simulink model "VEHICLE_DYN_TRAIN"  (R2019b)
settings: Solver=ode4  StartTime=0.0  StopTime=150  FixedStep=0.01  RelTol=1e-3
model workspace (MAT data in the model file):
  ACCEL = [0 0.000975932898663 -0.0414538855996 0.0440661905922 -0.0484817487001 0.0392964510644 -0.0693895143615 0.0261566921783 -0.0586295561215 0.0249771458914 -0.0595081132089 0.0233316013131 ... (544 elements, 17x32)]
  A_mc = 0.000491
  CMD_BR = [0 0 0 0 0 0 0 0 0 0 0 0 ... (15001 elements, 15001x1)]
  CMD_MODE = [1 1 1 1 1 1 1 1 1 1 1 1 ... (15001 elements, 15001x1)]
  CMD_ST = [0 0 0 0 0 0 0 0 0 0 0 0 ... (15001 elements, 15001x1)]
  CMD_T = [0 0.01 0.02 0.03 0.04 0.05 0.06 0.07 0.08 0.09 0.1 0.11 ... (2001 elements, 1x2001)]
  CMD_TH = [0 0 0 0 0 0 0 0 0 0 0 0 ... (15001 elements, 15001x1)]
  CMD_TM = [0 0.01 0.02 0.03 0.04 0.05 0.06 0.07 0.08 0.09 0.1 0.11 ... (15001 elements, 15001x1)]
  CMD_U = [10 10 10 10 10 10 10 10 10 10 10 10 ... (2001 elements, 1x2001)]
  CMD_UX = [0.1 0.1 0.1 0.1 0.1 0.1 0.1 0.1 0.1 0.1 0.1 0.1 ... (15001 elements, 15001x1)]
  COMMAND = [0 0 0 0 0 0 0 0 0 0 0 0 ... (102 elements, 17x6)]
  C_q = 1.4e-06
  DATA_HMMWV : object (value not decoded)
  DATA_VESIM_CC_BRAKE : object (value not decoded)
  FORCE = [0 -4628.45620853 2357.84853747 -1841.82564621 -1727.75397473 1695.19792057 -1263.06335256 1524.31841051 -1649.98396845 -1537.1025145 -1335.96213703 1639.88309903 ... (493 elements, 17x29)]
  F_cf = 80
  F_cs = 138
  F_z = -50097.6
  Gain_v = 70
  J_wheel = 32
  K_vb = 1500
  Kp_rpm = 2.7013
  Kp_v = 30
  L3 = 10
  MIN_TH = 0
  M_sprung = 4672
  M_unsprung = 220
  M_unsprung_front = 220
  M_vehicle = 5112
  N2 = 0
  N3 = 0.01
  P = 36
  P_0 = 10670
  P_gain = 0.0006
  R_wheel = 0.4412
  SLIP = [0 -0.5 0.5 -0.5 -0.5 0.5 -0.5 0.5 -0.5 -0.5 -0.5 0.5 ... (136 elements, 17x8)]
  STATE = [0 4.33747954961e-06 -0.000147430460781 -3.72129119222e-05 -0.000284189368187 -0.000207128204422 -0.00055150808757 -0.000594561033148 -0.000967775941564 -0.00103412952076 -0.00143215770154 -0.00152470872631 ... (544 elements, 17x32)]
  STATES_INIT = [0 0 0.9902452 0 0 1.57079632679 0.01 0 0 0 0 0 ... (32 elements, 1x32)]
  SUSP = [0 -0.00875795294893 -0.00878173856984 -0.00830852863719 -0.00873591176348 -0.00870428588158 -0.00751721170558 -0.00851904716693 -0.00789923296531 -0.00838039895253 -0.00756270047902 -0.00866403364289 ... (612 elements, 17x36)]
  S_o = 3
  T2_r = 4
  TIRE = [0 0.0910654620457 -0.0936729683319 0.0717372732987 0.0513932148365 -0.0365035701266 -0.00739813929507 -0.0045484168787 0.0723881675257 0.0296400174207 -0.0169805208571 0.0207214713062 ... (408 elements, 17x24)]
  TIRELIFTOFF = [0 0 0 0 0 0 0 0 0 0 0 0 ... (17 elements, 17x1)]
  T_LENGTH = 2001
  T_STEP = 0.01
  T_STOP = 12.82
  T_TOTAL = 20
  Ti_rpm = 0.6464
  Ti_v = 2.5
  Tstop = [150 150 150 150 150 150 150 150 150 150 150 150 ... (15001 elements, 15001x1)]
  Tt_rpm = 0.0808
  Tt_v = 0.3125
  U_INIT = 0.01
  b = 170
  brake_Pw = [-3.96235801772 -3.96238075942 -0.895107722214 -0.895547395081 35.9159438465 72.7273668629 152.485661058 244.514654481 330.408495385 364.152342142 462.316700341 535.939857177 ... (40 elements, 40x1)]
  brake_V = [-1.14468402636e-08 6.09303685082e-09 2.9257815427e-07 6.31682445149e-07 8.18779962309e-07 1.05849711081e-06 1.41515318379e-06 1.67826507702e-06 1.8361367918e-06 2.02323385108e-06 2.22788040303e-06 2.46760304614e-06 ... (40 elements, 40x1)]
  diff_efficiency = 0.94
  diff_wRatio = 6.052
  diff_w_ratio = 3.56
  end_time = 140
  engine_inertia = 0.53
  fmin_mg = [42.75 43.31 51.6 64.3 73.65 71.1 72.7 72.36]
  fmin_mg_na = [42.79 42.79 42.79 42.79 42.79 42.79 42.79 42.79]
  g = -9.8
  g_motor_eff = 1
  gr_motor = 0
  i = 5
  mdot_fuel = [5e-06 1e-05 2e-05 3e-05 4e-05 5e-05 6e-05 7e-05 8e-05]
  ms2mph = 2.23694
  n_tire = 4
  no_cyl = 8
  num_points = 14000
  num_points_fast = 140000
  rpm0 = 83.7758040957
  rpm0_c = 1000
  rpm2rads = 0.10471975512
  rpm_e = [50 800 1000 1500 2000 2500 3000 3300]
  rpm_engine = [700 800 1000 1500 2000 2500 3000 3300]
  rpm_hi_idle = 3400
  rpm_idle = 750
  rpm_max_c = 3200
  rpm_rated = 3200
  start_time = 0
  time_step = 0.01
  time_step_fast = 0.001
  torque_engine = [9.767 15.303 12.411 -4.524 -12.214 -35.77 -70 -75.889 75.383 80.318 76.501 61.314 ... (72 elements, 8x9)]
  tout = [0 0.01 0.02 0.03 0.04 0.05 0.06 0.07 0.08 0.09 0.1 0.11 ... (17 elements, 17x1)]
  trq_scale = 0.46
values from neighbouring files (symbols this model uses):
  B = Ref(i:i+2,2)    [Calc_vref.m]    (also in Parameter_load.m = 0.1; VEHICLE_DYN_TRAIN_INIT.m = 0.25)
  Error_now = Error_now_array(end)    [RUN_SIMULATION_SHARED_NEW_POWERTRAIN.m]    (also in VEHICLE_DYN_TRAIN_INIT.m = 0)
  J = 0.075    [VEHICLE_DYN_TRAIN_INIT.m]
  K = 0.075    [VEHICLE_DYN_TRAIN_INIT.m]
  pid2tau_gain = 2.5    [VEHICLE_DYN_TRAIN_INIT.m]
  st_a_in = st_sc_out(end)    [RUN_SIMULATION_SHARED_NEW_POWERTRAIN.m]    (also in VEHICLE_DYN_TRAIN_INIT.m = 0)
  tau_a_in = tau_a_out(end)    [RUN_SIMULATION_SHARED_NEW_POWERTRAIN.m]    (also in VEHICLE_DYN_TRAIN_INIT.m = 0)
undefined symbols (not defined in the file or in its folder): adaptive_flag, autonomy_human_contain_gain, Bias_Distance, dt, error_lookuptable, human_autonomy_agreement_threshold, human_contain_min, human_response_dead_zone, human_torque_max, J_cal, kp_sc, model_lookuptable, Standard_Devices, steering_stable_threshold, UDP_Protocol, vdes, Xobs, Yobs
libraries: simulink x16, sldrtlib x3, dspstat3 x3, vrlib x2
(part 2 of 4)

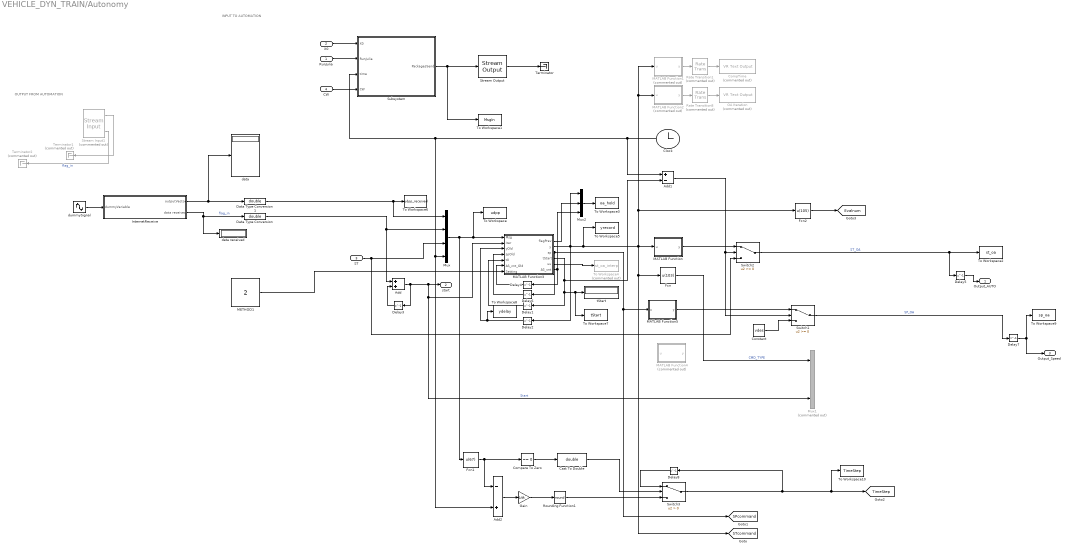
== system VEHICLE_DYN_TRAIN/Autonomy ==
  note: OUTPUT FROM AUTOMATION
  note: INPUT TO AUTOMATION
  RunJulia : Inport
  X0 : Inport  Port=2
  ST : Inport  Port=3
  CW : Inport  Port=4
  Add : Sum
  Add1 : Sum  Inputs=+-
  Add2 : Sum  Inputs=-+
  Cast To Double : DataTypeConversion  OutDataTypeStr=double
  Clock : Clock
      settings: Decimation=100
  CompTime : vrlib/VR Text Output  Commented=on  Ts=-1  ForceViewerOpen=off
      settings: SourceProductName=Simulink 3D Animation  SourceProductBaseCode=VR
  Compare To Zero : simulink/Logic and Bit Operations/Compare To Zero  relop===  OutDataTypeStr=boolean
  Constant : Constant  Value=vdes
  Data Type Conversion : DataTypeConversion  OutDataTypeStr=double
  Data Type Conversion1 : DataTypeConversion  OutDataTypeStr=double
  Delay{1,3..5,7..8} (6 alike) : Delay  DelayLength=1  InitialCondition=0  SampleTime=dt
  Delay2 : Delay  DelayLength=1  InitialCondition=zeros(110,1)  SampleTime=dt
  Delay6 : Delay  DelayLength=1  InitialCondition=zeros(110,1)  SampleTime=dt
  Fcn : Fcn  Expr=u(103)
  Fcn1 : Fcn  Expr=u(67)
  Fcn2 : Fcn  Expr=u(105)
  Gain : Gain  Gain=1/dt
  InternetReceive : Subsystem  mask(20-sim 4.6 S-Function block){}
      mask help:
      | This block is generated by the 20-sim Matlab Code Generator.
      |
      | * look under the mask to get information on the ports
      | * press Help for more detailed information
      | * the parameters of this block are:
      mask Help:
      | This block is generated by the 20-sim Matlab Code Generator<br>
      | The block parameters are:<br><blockquote></blockquote>
      | Generated at:<br>
      | <blockquote><b>date:  </b>June 14, 2017<br>
      | <b>time:  </b>4:16:43 PM<br></blockquote>
      | From the following 20-sim model:<br>
      | <blockquote><b>submodel:  </b>InternetServer<br>
      | <b>model:  </b>export to Simulink - UM<br>
      | <b>file:  </b>C:\Users\Tulga Ersal\Desktop\For Xueru\export to Simulink - UM.emx<br>
      | <b>experiment:  </b>C:\Users\Tulga Ersal\Desktop\For Xueru\export to Simulink - UM.emx<br></blockquote>
      | Using the following 20-sim license:<br>
      | <blockquote><b>user:  </b>The University of Michigan<br>
      | <b>from:  </b>20-sim 4.6 Student License<br>
      | <b>build: </b>4.6.1.6898<br></blockquote>
  MATLAB Function : MATLAB Function  TreatAsAtomicUnit=on
  MATLAB Function1 : MATLAB Function  Commented=on  TreatAsAtomicUnit=on
  MATLAB Function2 : MATLAB Function  Commented=on  TreatAsAtomicUnit=on
  MATLAB Function3 : MATLAB Function  TreatAsAtomicUnit=on
  MATLAB Function4 : MATLAB Function  Commented=on  TreatAsAtomicUnit=on
  MATLAB Function5 : MATLAB Function  TreatAsAtomicUnit=on
  METHOD1 : Constant  Value=2
  Mux : Mux
  Mux1 : Mux  Commented=on  Inputs=3
  Mux2 : Mux  Inputs=3
  OA Iteration : vrlib/VR Text Output  Commented=on  Ts=-1  ForceViewerOpen=off
      settings: SourceProductName=Simulink 3D Animation  SourceProductBaseCode=VR
  Rate Transition1 : RateTransition  Commented=on
  Rate Transition8 : RateTransition  Commented=on
  Rounding Function1 : Rounding  Operator=round
  Stream Input1 : sldrtlib/Stream Input  Commented=on  SampleTime=0.01  MaxMissedTicks=Inf  ShowMissedTicks=off  YieldWhenWaiting=off  DrvName=Standard_Devices/UDP_Protocol  DrvAddress=36881  DrvOptions=[0 12000 49 57 50 46 49 54 56 46 49 46 55 0 0 0 0 0 0 0 0 0 0 0 0 0 0 0 0 0 0 0 0 0 0 0 0 0 0 0 0 0 0 0 0 0 0 0 0 0 0 0 0 0 0 0 0 0 0 0 0 0 0 0 0 0 0 0 0 0 0 0 0 0 0 0 0 0 0 0 0 0 0 0 0 0 0 0 0 0 0 0 0 0 0 0 0 0 0 0 0 0 0 0 0 0 0 0 0 0 0 0 0 0 0 0 0 0 0 0 0 0 0 0 0 0 0 0 0 0 0 0 0 0 0 0 0 0 0 0 0 0 0 0 0 0 0 0 0 0 0 0 0 0 0 0 0 0 0 0 0 0 0 0 0 0 0 0 0 0 0 0 0 0 0 0 0 0 0 0 0 0 0 0 0 0 0 0 0 0 0 0 0 0 0 0 0 0 0 0 0 0 0 0 0 0 0 0 0 0 0 0 0 0 0 0 0 0 0 0 0 0 0 0 0 0 0 0 0 0 0 0 0 0 0 0 0 0 0 0 0 0 0 0 0 0 0 0 0 0 0 0 0 0 0 0]  DataTypes={'68*double'}  FormatString='%f,%f,%f,%f,%f,%f,%f,%f,%f,%f,%f,%f,%f,%f,%f,%f,%f,%f,%f,%f,%f,%f,%f,%f,%f,%f,%f,%f,%f,%f,%f,%f,%f,%f,%f,%f,%f,%f,%f,%f,%f,%f,%f,%f,%f,%f,%f,%f,%f,%f,%f,%f,%f,%f,%f,%f,%f,%f,%f,%f,%f,%f,%f,%f,%f,%f,%f,%f'  Terminator={ '\r', '\n' }  ShowReady=on  ShowError=off
      settings: AttributesFormatString=UDP Protocol [36881]  SourceProductName=Simulink Desktop Real-Time  SourceProductBaseCode=WT
  Stream Output : sldrtlib/Stream Output  SampleTime=0.01  MaxMissedTicks=Inf  ShowMissedTicks=on  YieldWhenWaiting=off  DrvName=Standard_Devices/UDP_Protocol  DrvAddress=36864  DrvOptions=[0 36880 49 57 50 46 49 54 56 46 49 46 55 0 0 0 0 0 0 0 0 0 0 0 0 0 0 0 0 0 0 0 0 0 0 0 0 0 0 0 0 0 0 0 0 0 0 0 0 0 0 0 0 0 0 0 0 0 0 0 0 0 0 0 0 0 0 0 0 0 0 0 0 0 0 0 0 0 0 0 0 0 0 0 0 0 0 0 0 0 0 0 0 0 0 0 0 0 0 0 0 0 0 0 0 0 0 0 0 0 0 0 0 0 0 0 0 0 0 0 0 0 0 0 0 0 0 0 0 0 0 0 0 0 0 0 0 0 0 0 0 0 0 0 0 0 0 0 0 0 0 0 0 0 0 0 0 0 0 0 0 0 0 0 0 0 0 0 0 0 0 0 0 0 0 0 0 0 0 0 0 0 0 0 0 0 0 0 0 0 0 0 0 0 0 0 0 0 0 0 0 0 0 0 0 0 0 0 0 0 0 0 0 0 0 0 0 0 0 0 0 0 0 0 0 0 0 0 0 0 0 0 0 0 0 0 0 0 0 0 0 0 0 0 0 0 0 0 0 0 0 0 0 0 0 0]  PortSizes=[23]  FormatString='%f %f %f %f %f %f %f %f %f %f %f %f %f %f %f %f %f %f %f %f %f %f %f \n'  ShowReady=off  ShowError=off  InitialValue=[]  FinalValue=[]
      settings: AttributesFormatString=UDP Protocol [36864]  SourceProductName=Simulink Desktop Real-Time  SourceProductBaseCode=WT
  Subsystem : Subsystem
  Switch1 : Switch
  Switch2 : Switch
  Switch3 : Switch  Criteria=u2 > Threshold
  Terminator : Terminator
  Terminator1 : Terminator  Commented=on
  Terminator2 : Terminator  Commented=on
  To Workspace : ToWorkspace  VariableName=udpp  SampleTime=-1
      settings: Save2DSignal=2-D array (concatenate along first dimension)
  To Workspace1 : ToWorkspace  VariableName=MsgIn  SampleTime=-1
  To Workspace10 : ToWorkspace  VariableName=TimeStep  SampleTime=-1
  To Workspace2 : ToWorkspace  VariableName=st_oa  SampleTime=-1
  To Workspace3 : ToWorkspace  VariableName=oa_hold  SampleTime=-1
  To Workspace4 : ToWorkspace  Commented=on  VariableName=st_oa_interp  SampleTime=-1
  To Workspace5 : ToWorkspace  VariableName=yrecord  SampleTime=-1
      settings: Save2DSignal=2-D array (concatenate along first dimension)
  To Workspace6 : ToWorkspace  VariableName=udpp_received  SampleTime=-1
      settings: Save2DSignal=2-D array (concatenate along first dimension)
  To Workspace7 : ToWorkspace  VariableName=tStart  SampleTime=-1
  To Workspace8 : ToWorkspace  VariableName=ydelay  SampleTime=-1
      settings: Save2DSignal=2-D array (concatenate along first dimension)
  To Workspace9 : ToWorkspace  VariableName=sp_oa  SampleTime=-1
  data : Display
  data received : Display
  dummySignal : Sin  SampleTime=0
  tStart : Display
  Output_AUTO : Outport  VectorParamsAs1DForOutWhenUnconnected=off
  start : Outport  Port=2  VectorParamsAs1DForOutWhenUnconnected=off
  Output_Speed : Outport  Port=3  VectorParamsAs1DForOutWhenUnconnected=off
  tag scope: Evalnum=global, SPcommand=global, STcommand=global, TimeStep=global
  wires:
  Data Type Conversion1/1 -> Mux/1, To Workspace6/1
  MATLAB Function3/5(uu) -> To Workspace4/1
  MATLAB Function/1(y) -> Switch2/1
  Add1/1 -> Switch1/2, Switch2/2
  Add/1 -> Delay3/1, Mux1/3, MATLAB Function3/2(iter), start/1  "Start"
  Subsystem/1(PackagesSend) -> Stream Output/1, To Workspace1/1
  Rate Transition8/1 -> OA Iteration/1
  MATLAB Function3/6(AS_cnt) -> Mux2/3, Delay4/1
  Fcn/1 -> Mux1/1  "CMD_TYPE"
  MATLAB Function2/1(y) -> Rate Transition8/1
  Rate Transition1/1 -> CompTime/1
  MATLAB Function3/4(tStart) -> Add1/2, Delay1/1, To Workspace7/1, tStart/1
  Delay4/1 -> MATLAB Function3/6(AS_cnt_Old)
  RunJulia/1 -> Subsystem/2(RunJulia)
  MATLAB Function3/1(flagPrev) -> Mux2/2
  Delay1/1 -> MATLAB Function3/5(t0)
  Data Type Conversion/1 -> Add/1, Mux/2
  Mux2/1 -> To Workspace3/1
  METHOD1/1 -> MATLAB Function3/7(Setting)
  Delay3/1 -> Add/2
  Switch2/1 -> Delay5/1, To Workspace2/1  "ST_OA"
  X0/1 -> Subsystem/1(X0)
  MATLAB Function1/1(y) -> Rate Transition1/1
  Delay2/1 -> To Workspace8/1, MATLAB Function3/3(yOld)
  Stream Output/1 -> Terminator/1
  ST/1 -> Switch2/3, Mux/3
  Delay5/1 -> Output_AUTO/1
  CW/1 -> Subsystem/4(CW)
  Delay6/1 -> MATLAB Function3/4(spOld)
  MATLAB Function5/1(y) -> Switch1/1
  Constant/1 -> Switch1/3
  Switch1/1 -> Delay7/1  "SP_OA"
  Delay7/1 -> Output_Speed/1, To Workspace9/1
  Delay8/1 -> Switch3/1
  Add2/1 -> Gain/1
  MATLAB Function3/3(sp) -> MATLAB Function5/1(u), [SPcommand], Delay6/1
  Cast To Double/1 -> Switch3/2
  Compare To Zero/1 -> Cast To Double/1
  Clock/1 -> Subsystem/3(time), Add2/2, Mux/4, Add1/1
  Mux/1 -> Fcn1/1, To Workspace/1, MATLAB Function3/1(Msg)
  Fcn1/1 -> Compare To Zero/1, Add2/1
  MATLAB Function3/2(y) -> Delay2/1, To Workspace5/1, [STcommand], Fcn/1, MATLAB Function1/1(u), MATLAB Function2/1(u), Fcn2/1, MATLAB Function/1(u), Mux2/1
  Fcn2/1 -> [Evalnum]
  Gain/1 -> Rounding Function1/1
  Rounding Function1/1 -> Switch3/3
  Switch3/1 -> [TimeStep], To Workspace10/1, Delay8/1
  InternetReceive/2(data received) -> Data Type Conversion/1, data received/1  "flag_in"
  dummySignal/1 -> InternetReceive/1(dummyVariable)
  InternetReceive/1(outputVector) -> Data Type Conversion1/1, data/1
  Stream Input1/1 -> Terminator1/1
  Stream Input1/2 -> Terminator2/1  "flag_in"

== system VEHICLE_DYN_TRAIN/Cognitive Workload Estimator ==
  Clock : Clock  Commented=on
  Constant : Constant
  Constant2 : Constant  Value=0.05
  Constant4 : Constant  Value=50
  Constant5 : Constant  Value=80
  MATLAB Function : MATLAB Function  Commented=on  TreatAsAtomicUnit=on
  Switch : Switch  Criteria=u2 > Threshold  Threshold=0.1
  Terminator : Terminator
  Workload : Outport  VectorParamsAs1DForOutWhenUnconnected=off
  wires:
  Clock/1 -> MATLAB Function/1(u)
  Constant2/1 -> Switch/2
  Constant5/1 -> Switch/1
  Constant4/1 -> Switch/3
  Switch/1 -> Workload/1
  Constant/1 -> Terminator/1

== system VEHICLE_DYN_TRAIN/Communication Unit ==
  HI : Inport
  Vehicle States : Inport  Port=2
  Speed : Inport  Port=3
  Demux : Demux
  Mux : Mux  Inputs=6
  Stream Output : sldrtlib/Stream Output  SampleTime=0.01  MaxMissedTicks=Inf  ShowMissedTicks=on  YieldWhenWaiting=off  DrvName=Standard_Devices/UDP_Protocol  DrvAddress=10001  DrvOptions=[0 10002 49 57 50 46 49 54 56 46 49 46 55 0 0 0 0 0 0 0 0 0 0 0 0 0 0 0 0 0 0 0 0 0 0 0 0 0 0 0 0 0 0 0 0 0 0 0 0 0 0 0 0 0 0 0 0 0 0 0 0 0 0 0 0 0 0 0 0 0 0 0 0 0 0 0 0 0 0 0 0 0 0 0 0 0 0 0 0 0 0 0 0 0 0 0 0 0 0 0 0 0 0 0 0 0 0 0 0 0 0 0 0 0 0 0 0 0 0 0 0 0 0 0 0 0 0 0 0 0 0 0 0 0 0 0 0 0 0 0 0 0 0 0 0 0 0 0 0 0 0 0 0 0 0 0 0 0 0 0 0 0 0 0 0 0 0 0 0 0 0 0 0 0 0 0 0 0 0 0 0 0 0 0 0 0 0 0 0 0 0 0 0 0 0 0 0 0 0 0 0 0 0 0 0 0 0 0 0 0 0 0 0 0 0 0 0 0 0 0 0 0 0 0 0 0 0 0 0 0 0 0 0 0 0 0 0 0 0 0 0 0 0 0 0 0 0 0 0 0 0 0 0 0 0 0]  PortSizes=[6]  FormatString='%f %f %f %f %f %f\n'  ShowReady=off  ShowError=off  InitialValue=[]  FinalValue=[]
      settings: AttributesFormatString=UDP Protocol [10001]  SourceProductName=Simulink Desktop Real-Time  SourceProductBaseCode=WT
  Terminator : Terminator
  wires:
  Stream Output/1 -> Terminator/1
  Demux/4 -> Mux/4
  Vehicle States/1 -> Demux/1
  Demux/3 -> Mux/3
  Demux/2 -> Mux/2
  Demux/1 -> Mux/1
  HI/1 -> Mux/5
  Mux/1 -> Stream Output/1
  Speed/1 -> Mux/6

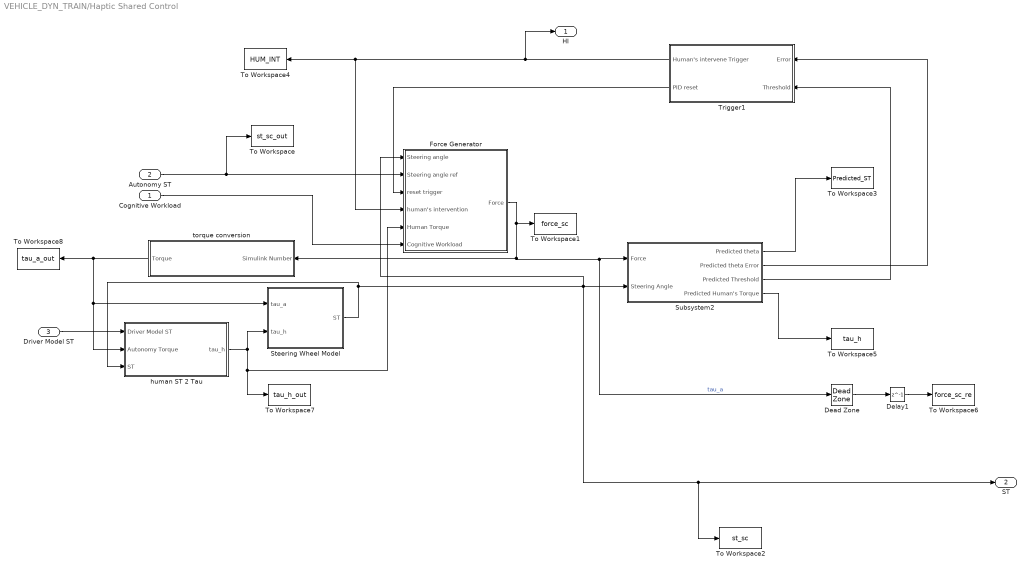
== system VEHICLE_DYN_TRAIN/Haptic Shared Control ==
  Cognitive Workload : Inport
  Autonomy ST : Inport  Port=2
  Driver Model ST : Inport  Port=3
  Dead Zone : DeadZone  LowerValue=F_f_n  UpperValue=F_f_p  SaturateOnIntegerOverflow=on
  Delay1 : Delay  DelayLength=1
  Force Generator : Subsystem
  Steering Wheel Model : Subsystem
  Subsystem2 : Subsystem
  To Workspace : ToWorkspace  VariableName=st_sc_out  SampleTime=-1
  To Workspace1 : ToWorkspace  VariableName=force_sc  SampleTime=-1
  To Workspace2 : ToWorkspace  VariableName=st_sc  SampleTime=-1
  To Workspace3 : ToWorkspace  VariableName=Predicted_ST  SampleTime=-1
  To Workspace4 : ToWorkspace  VariableName=HUM_INT  SampleTime=-1
  To Workspace5 : ToWorkspace  VariableName=tau_h  SampleTime=-1
  To Workspace6 : ToWorkspace  VariableName=force_sc_re  SampleTime=-1
  To Workspace7 : ToWorkspace  VariableName=tau_h_out  SampleTime=-1
  To Workspace8 : ToWorkspace  VariableName=tau_a_out  SampleTime=-1
  Trigger1 : Subsystem
  human ST 2 Tau : Subsystem
  torque conversion : Subsystem
  HI : Outport  VectorParamsAs1DForOutWhenUnconnected=off
  ST : Outport  Port=2  VectorParamsAs1DForOutWhenUnconnected=off
  wires:
  Subsystem2/1(Predicted theta) -> To Workspace3/1
  Cognitive Workload/1 -> Force Generator/6(Cognitive Workload)
  Trigger1/1(Human's intervene Trigger) -> HI/1, Force Generator/4(human's intervention), To Workspace4/1
  Subsystem2/2(Predicted theta Error) -> Trigger1/1(Error)
  Subsystem2/3(Predicted Threshold) -> Trigger1/2(Threshold)
  Trigger1/2(PID reset) -> Force Generator/3(reset trigger)
  Dead Zone/1 -> Delay1/1
  Subsystem2/4(Predicted Human's Torque) -> To Workspace5/1
  Delay1/1 -> To Workspace6/1
  Driver Model ST/1 -> human ST 2 Tau/1(Driver Model ST)
  Force Generator/1(Force) -> torque conversion/1(Simulink Number), Subsystem2/1(Force), Dead Zone/1, To Workspace1/1  "tau_a"
  Autonomy ST/1 -> To Workspace/1, Force Generator/2(Steering angle ref)
  torque conversion/1(Torque) -> human ST 2 Tau/2(Autonomy Torque), Steering Wheel Model/1(tau_a), To Workspace8/1
  human ST 2 Tau/1(tau_h) -> Force Generator/5(Human Torque), To Workspace7/1, Steering Wheel Model/2(tau_h)
  Steering Wheel Model/1(ST) -> human ST 2 Tau/3(ST), ST/1, To Workspace2/1, Subsystem2/2(Steering Angle), Force Generator/1(Steering angle)

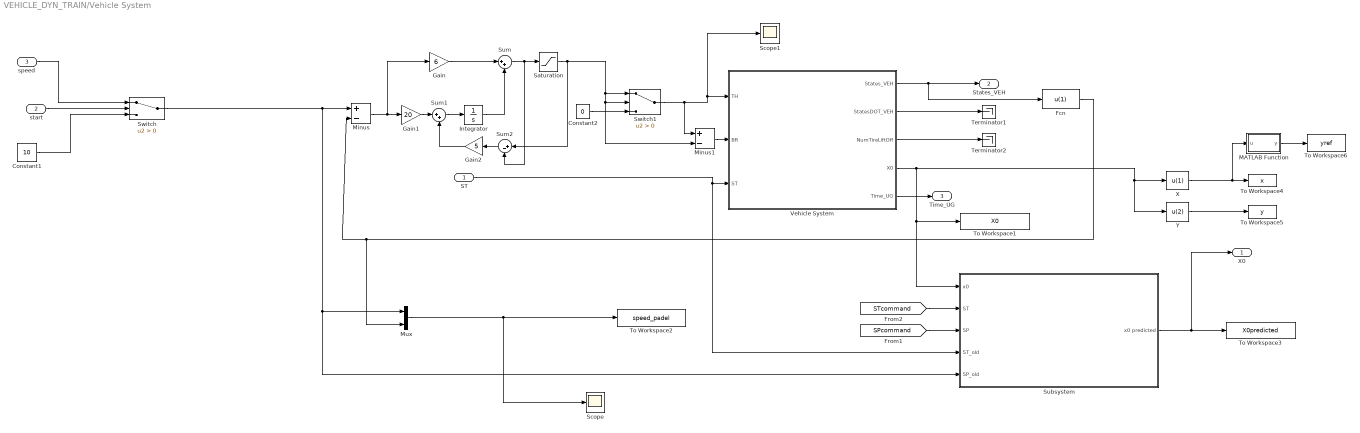
== system VEHICLE_DYN_TRAIN/Vehicle System ==
  ST : Inport
  start : Inport  Port=2
  speed : Inport  Port=3
  Constant1 : Constant  Value=10  SampleTime=dt
  Constant2 : Constant  Value=0  SampleTime=dt
  Fcn : Fcn  Expr=u(1)
  Gain : Gain  Gain=6
  Gain1 : Gain  Gain=20
  Gain2 : Gain  Gain=5
  Integrator : Integrator
  MATLAB Function : MATLAB Function  TreatAsAtomicUnit=on
  Minus : Sum  Inputs=+-
  Minus1 : Sum  Inputs=+-
  Mux : Mux  Inputs=2
  Saturation : Saturate  UpperLimit=1  LowerLimit=-1
  Scope : Scope
  Scope1 : Scope
  Subsystem : Subsystem
  Sum : Sum  Inputs=|++
  Sum1 : Sum  Inputs=|++
  Sum2 : Sum  Inputs=|+-
  Switch : Switch  Criteria=u2 > Threshold
  Switch1 : Switch  Criteria=u2 > Threshold
  Terminator1 : Terminator
  Terminator2 : Terminator
  To Workspace1 : ToWorkspace  VariableName=X0  SampleTime=-1
  To Workspace2 : ToWorkspace  VariableName=speed_padel  SampleTime=-1
  To Workspace3 : ToWorkspace  VariableName=X0predicted  SampleTime=-1
  To Workspace4 : ToWorkspace  VariableName=x  SampleTime=-1
  To Workspace5 : ToWorkspace  VariableName=y  SampleTime=-1
  To Workspace6 : ToWorkspace  VariableName=yref  SampleTime=-1
  Vehicle System : Subsystem
  X : Fcn  Expr=u(1)
  Y : Fcn  Expr=u(2)
  X0 : Outport  VectorParamsAs1DForOutWhenUnconnected=off
  States_VEH : Outport  Port=2  VectorParamsAs1DForOutWhenUnconnected=off
  Time_UG : Outport  Port=3  VectorParamsAs1DForOutWhenUnconnected=off
  wires:
  ST/1 -> Subsystem/4(ST_old), Vehicle System/3(ST)
  Vehicle System/1(States_VEH) -> Fcn/1, States_VEH/1
  Vehicle System/2(StatesDOT_VEH) -> Terminator1/1
  Vehicle System/3(NumTireLiftOff) -> Terminator2/1
  Fcn/1 -> Mux/2, Minus/2
  Minus/1 -> Gain1/1, Gain/1
  Gain/1 -> Sum/1
  Gain1/1 -> Sum1/1
  Sum1/1 -> Integrator/1
  Integrator/1 -> Sum/2
  Gain2/1 -> Sum1/2
  Sum2/1 -> Gain2/1
  Sum/1 -> Saturation/1, Sum2/2
  Saturation/1 -> Minus1/2, Switch1/2, Switch1/1, Sum2/1
  Switch1/1 -> Scope1/1, Vehicle System/1(TH), Minus1/1
  Constant2/1 -> Switch1/3
  Minus1/1 -> Vehicle System/2(BR)
  speed/1 -> Switch/1
  Constant1/1 -> Switch/3
  start/1 -> Switch/2
  Mux/1 -> Scope/1, To Workspace2/1
  Switch/1 -> Subsystem/5(SP_old), Mux/1, Minus/1
  [STcommand] -> Subsystem/2(ST)
  [SPcommand] -> Subsystem/3(SP)
  Subsystem/1(x0 predicted) -> X0/1, To Workspace3/1
  X/1 -> MATLAB Function/1(u), To Workspace4/1
  MATLAB Function/1(y) -> To Workspace6/1
  Y/1 -> To Workspace5/1
  Vehicle System/4(X0) -> Subsystem/1(x0), To Workspace1/1, Y/1, X/1
  Vehicle System/5(Time_UG) -> Time_UG/1

== system VEHICLE_DYN_TRAIN/Autonomy/InternetReceive ==
  dummyVariable : Inport
  Demux : Demux  Outputs=[1 -1]
  S-Function : S-Function  FunctionName=InternetServer  SFunctionDeploymentMode=off  EnableBusSupport=off
  outputVector : Outport  VectorParamsAs1DForOutWhenUnconnected=off
  data received : Outport  Port=2  VectorParamsAs1DForOutWhenUnconnected=off
  wires:
  dummyVariable/1 -> S-Function/1
  S-Function/1 -> Demux/1
  Demux/1 -> data received/1
  Demux/2 -> outputVector/1

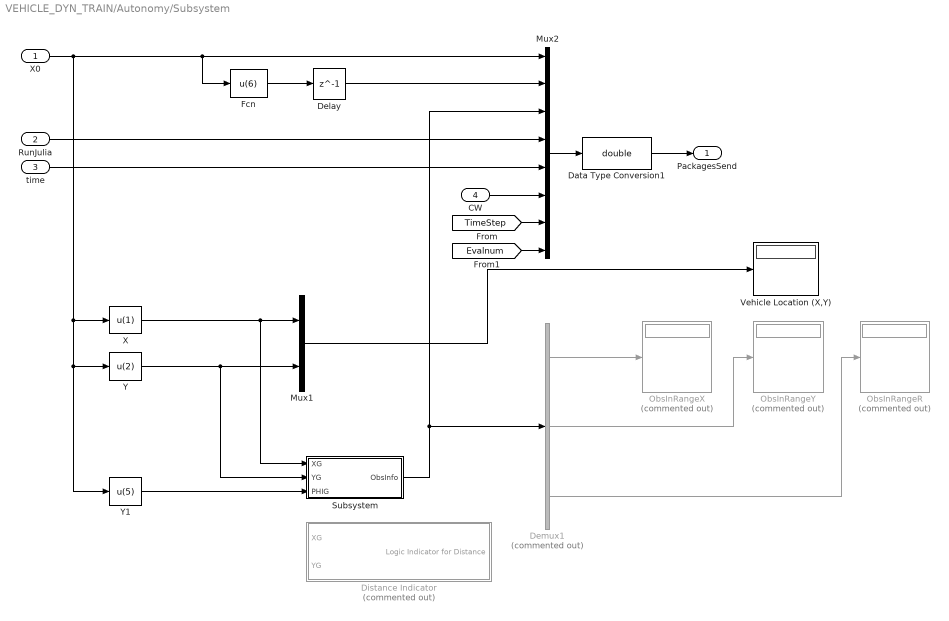
== system VEHICLE_DYN_TRAIN/Autonomy/Subsystem ==
  X0 : Inport
  RunJulia : Inport  Port=2
  time : Inport  Port=3
  CW : Inport  Port=4
  Data Type Conversion1 : DataTypeConversion  OutDataTypeStr=double
  Delay : Delay  DelayLength=1  InitialCondition=0  SampleTime=dt
  Demux1 : Demux  Commented=on  Outputs=[3 3 3]
  Distance Indicator : Subsystem  Commented=on
  Fcn : Fcn  Expr=u(6)
  Mux1 : Mux  Inputs=2
  Mux2 : Mux  Inputs=8
  ObsInRangeR : Display  Commented=on
  ObsInRangeX : Display  Commented=on
  ObsInRangeY : Display  Commented=on
  Subsystem : Subsystem
  Vehicle Location (X,Y) : Display
  X : Fcn  Expr=u(1)
  Y : Fcn  Expr=u(2)
  Y1 : Fcn  Expr=u(5)
  PackagesSend : Outport  VectorParamsAs1DForOutWhenUnconnected=off
  wires:
  Data Type Conversion1/1 -> PackagesSend/1
  Mux2/1 -> Data Type Conversion1/1
  X0/1 -> Y1/1, Y/1, X/1, Fcn/1, Mux2/1
  Y/1 -> Subsystem/2(YG), Mux1/2
  Subsystem/1(ObsInfo) -> Mux2/3, Demux1/1
  Mux1/1 -> Vehicle Location (X,Y)/1
  Demux1/1 -> ObsInRangeX/1
  Demux1/2 -> ObsInRangeY/1
  Demux1/3 -> ObsInRangeR/1
  time/1 -> Mux2/5
  RunJulia/1 -> Mux2/4
  Delay/1 -> Mux2/2
  Fcn/1 -> Delay/1
  Y1/1 -> Subsystem/3(PHIG)
  X/1 -> Subsystem/1(XG), Mux1/1
  CW/1 -> Mux2/6
  [TimeStep] -> Mux2/7
  [Evalnum] -> Mux2/8

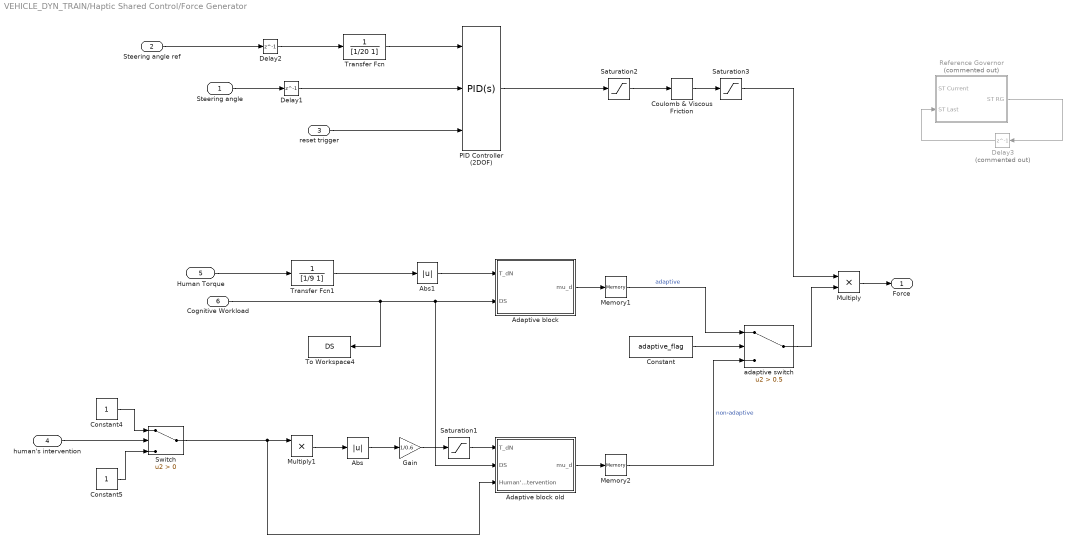
== system VEHICLE_DYN_TRAIN/Haptic Shared Control/Force Generator ==
  Steering angle : Inport
  Steering angle ref : Inport  Port=2
  reset trigger : Inport  Port=3
  human's intervention : Inport  Port=4
  Human Torque : Inport  Port=5
  Cognitive Workload : Inport  Port=6
  Abs : Abs
  Abs1 : Abs
  Adaptive block : Subsystem
  Adaptive block old : Subsystem
  Constant : Constant  Value=adaptive_flag
  Constant4 : Constant
  Constant5 : Constant
  Coulomb & Viscous Friction : simulink/Discontinuities/Coulomb & Viscous Friction  offset=0.12  gain=1
      settings: SourceProductName=Simulink
  Delay1 : Delay  DelayLength=1
  Delay2 : Delay  DelayLength=1
  Delay3 : Delay  Commented=on  DelayLength=1
  Gain : Gain  Gain=1/0.6
  Memory1 : Memory
  Memory2 : Memory
  Multiply : Product
  Multiply1 : Product
  PID Controller (2DOF) : simulink/Continuous/PID Controller (2DOF)  Controller=PID  Form=Parallel  TimeDomain=Continuous-time  SampleTime=-1  IntegratorMethod=Forward Euler  FilterMethod=Forward Euler  ControllerParametersSource=internal  P=20  I=10  D=0.75  UseFilter=on  N=100  b=1  c=1  TunerSelectOption=Transfer Function Based (PID Tuner App)  ZeroCross=off  InitialConditionSource=internal  InitialConditionForIntegrator=0  InitialConditionForFilter=0  DifferentiatorICPrevScaledInput=0  ExternalReset=rising  TrackingMode=off  Kt=1  LimitOutput=off  UpperSaturationLimit=inf  LowerSaturationLimit=-inf  LinearizeAsGain=on  AntiWindupMode=none  Kb=1  POutMin=[]  POutMax=[]  IOutMin=[]  IOutMax=[]  DOutMin=[]  DOutMax=[]  NOutMin=[]  NOutMax=[]  bOutMin=[]  bOutMax=[]  cOutMin=[]  cOutMax=[]  SumOutMin=[]  SumOutMax=[]  SaturationOutMin=[]  SaturationOutMax=[]  PParamMin=[]  PParamMax=[]  IParamMin=[]  IParamMax=[]  DParamMin=[]  DParamMax=[]  NParamMin=[]  NParamMax=[]  bParamMin=[]  bParamMax=[]  cParamMin=[]  cParamMax=[]  KbParamMin=[]  KbParamMax=[]  KtParamMin=[]  KtParamMax=[]  KbOutMin=[]  KbOutMax=[]  KtOutMin=[]  KtOutMax=[]  IntegratorOutMin=[]  IntegratorOutMax=[]  FilterOutMin=[]  FilterOutMax=[]  SumI1OutMin=[]  SumI1OutMax=[]  SumI2OutMin=[]  SumI2OutMax=[]  SumI3OutMin=[]  SumI3OutMax=[]  SumI4OutMin=[]  SumI4OutMax=[]  SumDOutMin=[]  SumDOutMax=[]  Sum1OutMin=[]  Sum1OutMax=[]  Sum2OutMin=[]  Sum2OutMax=[]  Sum3OutMin=[]  Sum3OutMax=[]  DifferentiatorOutMin=[]  DifferentiatorOutMax=[]  FilterDiffOutCoefMin=[]  FilterDiffOutCoefMax=[]  ReciprocalOutMin=[]  ReciprocalOutMax=[]  SumDenOutMin=[]  SumDenOutMax=[]  SumNumOutMin=[]  SumNumOutMax=[]  DivideOutMin=[]  DivideOutMax=[]  IntegratorContinuousStateAttributes=''  IntegratorStateMustResolveToSignalObject=off  IntegratorRTWStateStorageClass=Auto  FilterContinuousStateAttributes=''  FilterStateMustResolveToSignalObject=off  FilterRTWStateStorageClass=Auto  ParallelPVariant=InternalParameters  IdealPVariant=Disabled  IVariant=InternalParameters  DVariant=InternalParameters  bVariant=InternalParameters  cVariant=InternalParameters  IntegratorVariant=Continuous  SatVariant=Disabled  AWVariant=Passthrough  PCopyVariant=Disabled  TRVariant=Disabled  FdbkBlocksVariant=Forward  IdealPFdbkVariant=Disabled  SatFdbkVariant=Disabled  DerivativeFilterVariant=ContFilter  NVariant=InternalParameters  NCopyVariant=Disabled  FilterICVariant=InternalICsFilter  IntegratorICVariant=InternalICs  ExternalResetVariant=ExternalReset  TRSumVariant=Passthrough  SumFdbkVariant=Disabled  SumVariant=Sum_PID
  Reference Governor : Subsystem  Commented=on
  Saturation1 : Saturate  UpperLimit=1  LowerLimit=0
  Saturation2 : Saturate  UpperLimit=0.59  LowerLimit=-0.59
  Saturation3 : Saturate  UpperLimit=0.59  LowerLimit=-0.59
  Switch : Switch  Criteria=u2 > Threshold
  To Workspace4 : ToWorkspace  VariableName=DS  SampleTime=-1
  Transfer Fcn : TransferFcn  Denominator=[1/20 1]
  Transfer Fcn1 : TransferFcn  Denominator=[1/9 1]
  adaptive switch : Switch  Criteria=u2 > Threshold  Threshold=0.5
  Force : Outport  VectorParamsAs1DForOutWhenUnconnected=off
  wires:
  Steering angle/1 -> Delay1/1
  Delay1/1 -> PID Controller (2DOF)/2
  Saturation2/1 -> Coulomb & Viscous Friction/1
  PID Controller (2DOF)/1 -> Saturation2/1
  Coulomb & Viscous Friction/1 -> Saturation3/1
  Steering angle ref/1 -> Delay2/1
  Saturation3/1 -> Multiply/1
  Multiply/1 -> Force/1
  Adaptive block old/1(mu_d) -> Memory2/1
  Gain/1 -> Saturation1/1
  Abs/1 -> Gain/1
  Saturation1/1 -> Adaptive block old/1(T_dN)
  Switch/1 -> Adaptive block old/3(Human's intervention), Multiply1/1
  Multiply1/1 -> Abs/1
  reset trigger/1 -> PID Controller (2DOF)/3
  Reference Governor/1(ST RG) -> Delay3/1
  Delay3/1 -> Reference Governor/2(ST Last)
  Delay2/1 -> Transfer Fcn/1
  Transfer Fcn/1 -> PID Controller (2DOF)/1
  Constant4/1 -> Switch/1
  Constant5/1 -> Switch/3
  human's intervention/1 -> Switch/2
  Adaptive block/1(mu_d) -> Memory1/1
  Cognitive Workload/1 -> To Workspace4/1, Adaptive block old/2(DS), Adaptive block/2(DS)
  Abs1/1 -> Adaptive block/1(T_dN)
  Human Torque/1 -> Transfer Fcn1/1
  Memory1/1 -> adaptive switch/1  "adaptive"
  Memory2/1 -> adaptive switch/3  "non-adaptive"
  Transfer Fcn1/1 -> Abs1/1
  adaptive switch/1 -> Multiply/2
  Constant/1 -> adaptive switch/2

== system VEHICLE_DYN_TRAIN/Haptic Shared Control/Steering Wheel Model ==
  tau_a : Inport
  tau_h : Inport  Port=2
  Constant : Constant  Value=0
  Drag1 : Gain  Gain=B
  Gain : Gain  Gain=0.1
  Integrator1 : Integrator
  Integrator2 : Integrator
  Moment of Inertia1 : Gain  Gain=1/J
  Stiffness : Gain  Gain=K
  Sum : Sum  Inputs=|++
  Sum3 : Sum  Inputs=|+-
  Sum5 : Sum  Inputs=|++
  Terminator : Terminator
  ST : Outport  VectorParamsAs1DForOutWhenUnconnected=off
  wires:
  Sum/1 -> Sum3/1  "tau_in"
  Sum5/1 -> Sum3/2
  Drag1/1 -> Sum5/1
  Integrator2/1 -> Stiffness/1, Gain/1  "theta"
  Integrator1/1 -> Drag1/1, Integrator2/1  "omega"
  Moment of Inertia1/1 -> Integrator1/1  "omega_dot"
  Sum3/1 -> Moment of Inertia1/1
  Stiffness/1 -> Sum5/2
  Gain/1 -> ST/1
  tau_a/1 -> Sum/2  "tau_a"
  Constant/1 -> Terminator/1
  tau_h/1 -> Sum/1

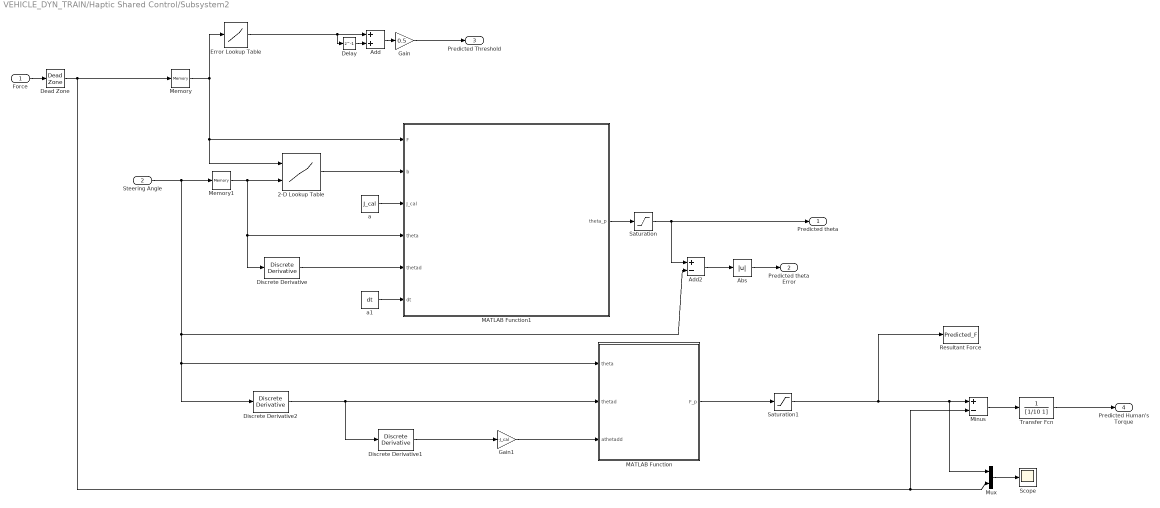
== system VEHICLE_DYN_TRAIN/Haptic Shared Control/Subsystem2 ==
  Force : Inport
  Steering Angle : Inport  Port=2
  2-D Lookup Table : Lookup_n-D  BreakpointsForDimension1=model_lookuptable.Breakpoints_row  BreakpointsForDimension2=model_lookuptable.Breakpoints_column  Table=model_lookuptable.Tabledata  InternalRulePriority=Speed  RndMeth=Simplest  InputSameDT=on
  Abs : Abs
  Add : Sum
  Add2 : Sum  Inputs=+-
  Dead Zone : DeadZone  LowerValue=F_f_n  UpperValue=F_f_p  SaturateOnIntegerOverflow=on
  Delay : Delay  DelayLength=1
  Discrete Derivative : simulink/Discrete/Discrete Derivative  gainval=1.0  ICPrevScaledInput=0.0  OutMin=[]  OutMax=[]  OutDataType=fixdt(1, 16)  OutScaling=2^-10  DoSatur=off
  Discrete Derivative1 : simulink/Discrete/Discrete Derivative  gainval=1.0  ICPrevScaledInput=0.0  OutMin=[]  OutMax=[]  OutDataType=fixdt(1, 16)  OutScaling=2^-10  DoSatur=off
  Discrete Derivative2 : simulink/Discrete/Discrete Derivative  gainval=1.0  ICPrevScaledInput=0.0  OutMin=[]  OutMax=[]  OutDataType=fixdt(1, 16)  OutScaling=2^-10  DoSatur=off
  Error Lookup Table : Lookup_n-D  NumberOfTableDimensions=1  BreakpointsForDimension1=error_lookuptable.Breakpoints  Table=error_lookuptable.Tabledata  InternalRulePriority=Speed  RndMeth=Simplest  InputSameDT=on
  Gain : Gain  Gain=0.5
  Gain1 : Gain  Gain=-J_cal
  MATLAB Function : MATLAB Function  TreatAsAtomicUnit=on
  MATLAB Function1 : MATLAB Function  TreatAsAtomicUnit=on
  Memory : Memory
  Memory1 : Memory
  Minus : Sum  Inputs=+-
  Mux : Mux  Inputs=2
  Resultant Force : ToWorkspace  VariableName=Predicted_F  SampleTime=-1
  Saturation : Saturate  UpperLimit=9/180*pi  LowerLimit=-9/180*pi
  Saturation1 : Saturate  UpperLimit=0.4386  LowerLimit=-0.4228
  Scope : Scope
  Transfer Fcn : TransferFcn  Denominator=[1/10 1]
  a : Constant  Value=J_cal
  a1 : Constant  Value=dt
  Predicted theta : Outport  VectorParamsAs1DForOutWhenUnconnected=off
  Predicted theta Error : Outport  Port=2  VectorParamsAs1DForOutWhenUnconnected=off
  Predicted Threshold : Outport  Port=3  VectorParamsAs1DForOutWhenUnconnected=off
  Predicted Human's Torque : Outport  Port=4  VectorParamsAs1DForOutWhenUnconnected=off
  wires:
  Discrete Derivative/1 -> MATLAB Function1/5(thetad)
  Saturation/1 -> Add2/1, Predicted theta/1
  Discrete Derivative1/1 -> Gain1/1
  Force/1 -> Dead Zone/1
  Gain1/1 -> MATLAB Function/3(athetadd)
  MATLAB Function/1(F_p) -> Saturation1/1
  Saturation1/1 -> Mux/1, Minus/1, Resultant Force/1
  Add2/1 -> Abs/1
  Abs/1 -> Predicted theta Error/1
  a/1 -> MATLAB Function1/3(J_cal)
  2-D Lookup Table/1 -> MATLAB Function1/2(b)
  MATLAB Function1/1(theta_p) -> Saturation/1
  a1/1 -> MATLAB Function1/6(dt)
  Steering Angle/1 -> Memory1/1, Add2/2, MATLAB Function/1(theta), Discrete Derivative2/1
  Memory/1 -> MATLAB Function1/1(F), 2-D Lookup Table/1, Error Lookup Table/1
  Memory1/1 -> Discrete Derivative/1, MATLAB Function1/4(theta), 2-D Lookup Table/2
  Discrete Derivative2/1 -> Discrete Derivative1/1, MATLAB Function/2(thetad)
  Delay/1 -> Add/2
  Error Lookup Table/1 -> Delay/1, Add/1
  Add/1 -> Gain/1
  Gain/1 -> Predicted Threshold/1
  Minus/1 -> Transfer Fcn/1
  Dead Zone/1 -> Minus/2, Mux/2, Memory/1
  Mux/1 -> Scope/1
  Transfer Fcn/1 -> Predicted Human's Torque/1

== system VEHICLE_DYN_TRAIN/Haptic Shared Control/Trigger1 ==
  Error : Inport
  Threshold : Inport  Port=2
  Compare To Constant : simulink/Logic and Bit Operations/Compare To Constant  relop===  const=0  OutDataTypeStr=boolean
  Compare To Constant1 : simulink/Logic and Bit Operations/Compare To Constant  relop===  const=1  OutDataTypeStr=boolean
  Delay1 : Delay  DelayLength=1  InitialCondition=zeros(1,10)
  Delay2 : Delay  DelayLength=1  InitialCondition=0
  Delay3 : Delay  DelayLength=1  InitialCondition=0
  Delay4 : Delay  DelayLength=1  InitialCondition=zeros(1,20)
  Logical Operator : Logic  AllPortsSameDT=off  OutDataTypeStr=boolean
  MATLAB Function : MATLAB Function  TreatAsAtomicUnit=on
  Terminator : Terminator
  Human's intervene Trigger : Outport  VectorParamsAs1DForOutWhenUnconnected=off
  PID reset : Outport  Port=2  VectorParamsAs1DForOutWhenUnconnected=off
  wires:
  MATLAB Function/3(tr_vect) -> Delay4/1
  Delay4/1 -> MATLAB Function/3(tr_vect_old)
  MATLAB Function/4(trigger) -> Delay2/1, Compare To Constant/1, Human's intervene Trigger/1
  MATLAB Function/1(vect) -> Delay1/1
  Delay1/1 -> MATLAB Function/2(vect_old)
  Threshold/1 -> MATLAB Function/4(threshold)
  Error/1 -> MATLAB Function/1(u)
  Logical Operator/1 -> Delay3/1
  Compare To Constant1/1 -> Logical Operator/2
  Compare To Constant/1 -> Logical Operator/1
  Delay2/1 -> Compare To Constant1/1
  MATLAB Function/2(flag) -> Terminator/1
  Delay3/1 -> PID reset/1

== system VEHICLE_DYN_TRAIN/Haptic Shared Control/human ST 2 Tau ==
  Driver Model ST : Inport
  Autonomy Torque : Inport  Port=2
  ST : Inport  Port=3
  Constant : Constant  Value=tau_a_in
  Constant1 : Constant  Value=st_a_in
  Constant3 : Constant  Value=kp_sc
  Constant4 : Constant  Value=human_response_dead_zone
  Constant5 : Constant  Value=autonomy_human_contain_gain
  Constant6 : Constant  Value=human_autonomy_agreement_threshold
  Constant7 : Constant  Value=human_contain_min
  Constant8 : Constant  Value=Error_now
  Delay : Delay  DelayLength=1  InitialCondition=0
  Derivative : Derivative  CoefficientInTFapproximation=1
  MATLAB Function : MATLAB Function  TreatAsAtomicUnit=on
  Moving Average : dspstat3/Moving Average  Method=Sliding window  ForgettingFactorPort=off  SpecifyWindowLength=on  WindowLength=4  ForgettingFactor=0.9  SimulateUsing=Code generation
  Saturation : Saturate  UpperLimit=human_torque_max  LowerLimit=-human_torque_max
  Sum : Sum  Inputs=|+-
  Terminator1 : Terminator
  To Workspace2 : ToWorkspace  VariableName=diff_h_a1  SampleTime=-1
  tau_h : Outport  VectorParamsAs1DForOutWhenUnconnected=off
  wires:
  Saturation/1 -> tau_h/1
  MATLAB Function/1(tau_h) -> Saturation/1
  Derivative/1 -> Moving Average/1
  Sum/1 -> To Workspace2/1
  Constant5/1 -> MATLAB Function/5(k_c)
  Constant4/1 -> MATLAB Function/4(dead_zone)
  ST/1 -> Delay/1
  Constant7/1 -> MATLAB Function/7(human_contain)
  Delay/1 -> MATLAB Function/9(theta_st), Derivative/1
  Moving Average/1 -> MATLAB Function/8(omega_st)
  Constant6/1 -> MATLAB Function/6(threshold)
  Constant3/1 -> MATLAB Function/3(kp_sc)
  Constant1/1 -> Sum/2
  Driver Model ST/1 -> Sum/1, MATLAB Function/2(st_h)
  Constant/1 -> MATLAB Function/1(tau_a_in)
  Autonomy Torque/1 -> Terminator1/1
  Constant8/1 -> MATLAB Function/10(Error_now)

== system VEHICLE_DYN_TRAIN/Haptic Shared Control/torque conversion ==
  Simulink Number : Inport
  Constant : Constant  Value=0
  Delay : Delay  Commented=through  DelayLength=1
  Gain : Gain  Gain=pid2tau_gain
  Ground : Ground
  MATLAB Function : MATLAB Function  TreatAsAtomicUnit=on
  Moving Average : dspstat3/Moving Average  Method=Sliding window  ForgettingFactorPort=off  SpecifyWindowLength=on  WindowLength=5  ForgettingFactor=0.9  SimulateUsing=Code generation
  Sum : Sum  Inputs=|+-
  Sum1 : Sum  Inputs=|++
  Terminator : Terminator
  To Workspace9 : ToWorkspace  VariableName=tau_a_pred  SampleTime=-1
  memory 5 time step : Subsystem
  Torque : Outport  VectorParamsAs1DForOutWhenUnconnected=off
  wires:
  MATLAB Function/1(yout) -> To Workspace9/1, Moving Average/1  "tau_a_pred"
  memory 5 time step/1(Out) -> MATLAB Function/1(x1)
  Gain/1 -> Sum1/1
  Sum/1 -> Gain/1
  Constant/1 -> Sum1/2, Sum/2
  Delay/1 -> Torque/1
  Moving Average/1 -> Terminator/1
  Sum1/1 -> Delay/1
  Ground/1 -> memory 5 time step/1(In)
  Simulink Number/1 -> Sum/1

== system VEHICLE_DYN_TRAIN/Vehicle System/Subsystem ==
  x0 : Inport
  ST : Inport  Port=2
  SP : Inport  Port=3
  ST_old : Inport  Port=4
  SP_old : Inport  Port=5
  Constant : Constant  Value=dt
  Delay5 : Delay  DelayLength=1  InitialCondition=[zeros(103,1);1;zeros(6,1)]
  Delay6 : Delay  DelayLength=1  InitialCondition=[vdes*ones(103,1);1;zeros(6,1)]
  MATLAB Function2 : MATLAB Function  TreatAsAtomicUnit=on
  To Workspace2 : ToWorkspace  VariableName=STcommand  SampleTime=-1
  To Workspace3 : ToWorkspace  VariableName=SPcommand  SampleTime=-1
  To Workspace4 : ToWorkspace  VariableName=st_length  SampleTime=-1
  index : Fcn  Expr=u(104)
  x0 predicted : Outport  VectorParamsAs1DForOutWhenUnconnected=off
  wires:
  ST/1 -> Delay5/1
  x0/1 -> MATLAB Function2/1(X0)
  SP/1 -> Delay6/1
  Constant/1 -> MATLAB Function2/6(dt)
  index/1 -> MATLAB Function2/5(idx)
  [TimeStep] -> MATLAB Function2/4(time_step)
  MATLAB Function2/1(X0predicted) -> x0 predicted/1
  Delay5/1 -> To Workspace4/1, To Workspace2/1, index/1, MATLAB Function2/2(ST_length)
  Delay6/1 -> MATLAB Function2/3(SP_length), To Workspace3/1
  SP_old/1 -> MATLAB Function2/8(sp_old)
  ST_old/1 -> MATLAB Function2/7(st_old)

== system VEHICLE_DYN_TRAIN/Vehicle System/Vehicle System ==
  TH : Inport
  BR : Inport  Port=2
  ST : Inport  Port=3
  Add : Sum
  Constant : Constant  Value=Bias_Distance
  Derivative : Derivative
  Derivative1 : Derivative
  Hydraulic brake : Subsystem
  Mux : Mux  Inputs=2
  Mux1 : Mux  Inputs=8
  Mux2 : Mux
  Mux3 : Mux
  Powertrain1 : Subsystem
  Rate Transition : RateTransition
  Vehicle Model1 : Subsystem
  States_VEH : Outport  VectorParamsAs1DForOutWhenUnconnected=off
  StatesDOT_VEH : Outport  Port=2  VectorParamsAs1DForOutWhenUnconnected=off
  NumTireLiftOff : Outport  Port=3  VectorParamsAs1DForOutWhenUnconnected=off
  X0 : Outport  Port=4  VectorParamsAs1DForOutWhenUnconnected=off
  Time_UG : Outport  Port=5  VectorParamsAs1DForOutWhenUnconnected=off
  wires:
  Powertrain1/1(T shaft) -> Vehicle Model1/1(T_shaft)
  Vehicle Model1/1(w_shaft) -> Powertrain1/1(w shaft)
  Vehicle Model1/2(UG) -> Mux/2, Mux1/7, Mux2/1, Derivative/1
  Vehicle Model1/3(X) -> Mux1/1, Mux2/2
  Vehicle Model1/4(Y) -> Add/1, Mux2/3
  Vehicle Model1/5(PSI) -> Mux1/5, Derivative1/1, Mux2/4
  Vehicle Model1/8(YDOT) -> Mux3/3
  Vehicle Model1/7(XDOT) -> Mux3/2
  Mux3/1 -> StatesDOT_VEH/1
  Mux2/1 -> States_VEH/1
  Hydraulic brake/1(Brake torque) -> Vehicle Model1/2(Brake_cmd)
  Vehicle Model1/10(NumTireLiftOff) -> Rate Transition/1
  Rate Transition/1 -> NumTireLiftOff/1
  ST/1 -> Mux1/6, Vehicle Model1/3(Steering)
  Derivative/1 -> Mux3/1
  Derivative1/1 -> Mux3/4
  TH/1 -> Powertrain1/2(throttle)
  BR/1 -> Hydraulic brake/1(Brake command)
  Mux1/1 -> X0/1
  Vehicle Model1/9(PSIDOT) -> Mux1/4
  Vehicle Model1/6(UGDOT) -> Mux1/8
  Vehicle Model1/11(VG) -> Mux1/3
  Vehicle Model1/12(Time) -> Mux/1
  Mux/1 -> Time_UG/1
  Add/1 -> Mux1/2
  Constant/1 -> Add/2

== system VEHICLE_DYN_TRAIN/Autonomy/Subsystem/Distance Indicator ==
  XG : Inport
  YG : Inport  Port=2
  Cast To Double : DataTypeConversion  OutDataTypeStr=double
  Compare To Constant : simulink/Logic and Bit Operations/Compare To Constant  relop=>=  const=0.5  OutDataTypeStr=boolean
  Delay1 : Delay  DelayLength=1  InitialCondition=0  SampleTime=dt
  Subsystem1 : Subsystem
  To Workspace4 : ToWorkspace  VariableName=distance_var  SampleTime=-1
  Logic Indicator for Distance : Outport  VectorParamsAs1DForOutWhenUnconnected=off
  wires:
  XG/1 -> Subsystem1/1(XG)
  Subsystem1/2(X_init_update) -> Delay1/1
  YG/1 -> Subsystem1/2(YG)
  Subsystem1/1(DisInfo) -> To Workspace4/1, Compare To Constant/1
  Delay1/1 -> Subsystem1/3(X_init)
  Compare To Constant/1 -> Cast To Double/1
  Cast To Double/1 -> Logic Indicator for Distance/1

== system VEHICLE_DYN_TRAIN/Autonomy/Subsystem/Subsystem ==
  XG : Inport
  YG : Inport  Port=2
  PHIG : Inport  Port=3
  Compare To Constant : simulink/Logic and Bit Operations/Compare To Constant  relop=<  const=900  OutDataTypeStr=boolean
  Data Type Conversion : DataTypeConversion  OutDataTypeStr=double
  Fcn : Fcn  Expr=u(1)
  MATLAB Function : MATLAB Function  TreatAsAtomicUnit=on
  Mux : Mux  Inputs=3
  ObsR : Constant  Value=[1 1 1]  SampleTime=dt
  Saturation : Saturate  UpperLimit=900  LowerLimit=0
  Saturation1 : Saturate  UpperLimit=900  LowerLimit=0
  Xobs : Constant  Value=Xobs  SampleTime=dt
  Yobs : Constant  Value=Yobs  SampleTime=dt
  vdes : Constant  Value=vdes  SampleTime=dt
  ObsInfo : Outport  VectorParamsAs1DForOutWhenUnconnected=off
  tag scope: Obsinfo=global
  wires:
  Xobs/1 -> MATLAB Function/4(Xobs)
  Yobs/1 -> MATLAB Function/5(Yobs)
  XG/1 -> MATLAB Function/1(XG)
  YG/1 -> MATLAB Function/2(YG)
  PHIG/1 -> MATLAB Function/3(PHIG)
  MATLAB Function/1(Xobs_pass) -> Saturation/1
  Saturation/1 -> Fcn/1, Mux/1
  Saturation1/1 -> Mux/2
  Mux/1 -> ObsInfo/1
  ObsR/1 -> Mux/3
  MATLAB Function/2(Yobs_pass) -> Saturation1/1
  vdes/1 -> MATLAB Function/6(vdes)
  Compare To Constant/1 -> Data Type Conversion/1
  Data Type Conversion/1 -> [Obsinfo]
  Fcn/1 -> Compare To Constant/1

== system VEHICLE_DYN_TRAIN/Haptic Shared Control/Force Generator/Adaptive block ==
  T_dN : Inport
  DS : Inport  Port=2
  Gain2 : Gain  Gain=1/2
  Gain3 : Gain  Gain=0.6
  MATLAB Function : MATLAB Function  TreatAsAtomicUnit=on
  Saturation3 : Saturate  UpperLimit=1  LowerLimit=0
  To Workspace2 : ToWorkspace  VariableName=T_dN  SampleTime=-1
  To Workspace4 : ToWorkspace  VariableName=beta  SampleTime=-1
  mu_d : Outport  VectorParamsAs1DForOutWhenUnconnected=off
  wires:
  DS/1 -> MATLAB Function/2(sigma)
  MATLAB Function/1(y) -> mu_d/1, To Workspace4/1
  T_dN/1 -> To Workspace2/1, Gain2/1
  Gain2/1 -> Saturation3/1
  Gain3/1 -> MATLAB Function/1(T)
  Saturation3/1 -> Gain3/1

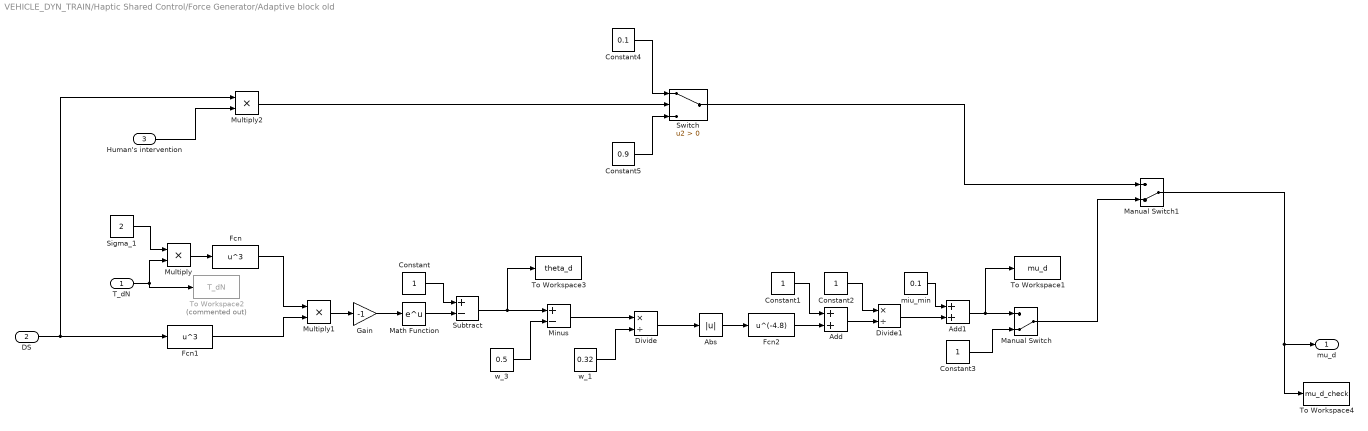
== system VEHICLE_DYN_TRAIN/Haptic Shared Control/Force Generator/Adaptive block old ==
  T_dN : Inport
  DS : Inport  Port=2
  Human's intervention : Inport  Port=3
  Abs : Abs
  Add : Sum
  Add1 : Sum
  Constant{,1..3} (4 alike) : Constant
  Constant4 : Constant  Value=0.1
  Constant5 : Constant  Value=0.9
  Divide : Product  Inputs=*/
  Divide1 : Product  Inputs=*/
  Fcn : Fcn  Expr=u^3
  Fcn1 : Fcn  Expr=u^3
  Fcn2 : Fcn  Expr=u^(-4.8)
  Gain : Gain  Gain=-1
  Manual Switch : ManualSwitch  CurrentSetting=0
  Manual Switch1 : ManualSwitch  CurrentSetting=0
  Math Function : Math  SaturateOnIntegerOverflow=on
  Minus : Sum  Inputs=+-
  Multiply : Product
  Multiply1 : Product
  Multiply2 : Product
  Sigma_1 : Constant  Value=2
  Subtract : Sum  Inputs=+-
  Switch : Switch  Criteria=u2 > Threshold
  To Workspace1 : ToWorkspace  VariableName=mu_d  SampleTime=-1
  To Workspace2 : ToWorkspace  Commented=on  VariableName=T_dN  SampleTime=-1
  To Workspace3 : ToWorkspace  VariableName=theta_d  SampleTime=-1
  To Workspace4 : ToWorkspace  VariableName=mu_d_check  SampleTime=-1
  miu_min : Constant  Value=0.1
  w_1 : Constant  Value=0.32
  w_3 : Constant  Value=0.5
  mu_d : Outport  VectorParamsAs1DForOutWhenUnconnected=off
  wires:
  Sigma_1/1 -> Multiply/1
  T_dN/1 -> Multiply/2, To Workspace2/1
  Multiply/1 -> Fcn/1
  Fcn/1 -> Multiply1/1
  Fcn1/1 -> Multiply1/2
  Multiply1/1 -> Gain/1
  Gain/1 -> Math Function/1
  Math Function/1 -> Subtract/2
  Constant/1 -> Subtract/1
  Subtract/1 -> Minus/1, To Workspace3/1
  w_3/1 -> Minus/2
  Minus/1 -> Divide/1
  w_1/1 -> Divide/2
  Divide/1 -> Abs/1
  Abs/1 -> Fcn2/1
  Fcn2/1 -> Add/2
  Constant1/1 -> Add/1
  Add/1 -> Divide1/2
  Constant2/1 -> Divide1/1
  Divide1/1 -> Add1/2
  miu_min/1 -> Add1/1
  Add1/1 -> Manual Switch/1, To Workspace1/1
  Manual Switch1/1 -> To Workspace4/1, mu_d/1
  Constant3/1 -> Manual Switch/2
  Manual Switch/1 -> Manual Switch1/2
  DS/1 -> Multiply2/1, Fcn1/1
  Human's intervention/1 -> Multiply2/2
  Multiply2/1 -> Switch/2
  Constant4/1 -> Switch/1
  Constant5/1 -> Switch/3
  Switch/1 -> Manual Switch1/1

== system VEHICLE_DYN_TRAIN/Haptic Shared Control/Force Generator/Reference Governor ==
  ST Current : Inport
  ST Last : Inport  Port=2
  MATLAB Function : MATLAB Function  TreatAsAtomicUnit=on
  ST RG : Outport  VectorParamsAs1DForOutWhenUnconnected=off
  wires:
  ST Current/1 -> MATLAB Function/1(ST_C)
  ST Last/1 -> MATLAB Function/2(ST_L)
  MATLAB Function/1(ST_RG) -> ST RG/1

== system VEHICLE_DYN_TRAIN/Haptic Shared Control/torque conversion/memory 5 time step ==
  In : Inport
  Memory{,1..4} (5 alike) : Memory
  Mux : Mux  Inputs=5
  Out : Outport  VectorParamsAs1DForOutWhenUnconnected=off
  wires:
  Memory3/1 -> Mux/2, Memory4/1
  Memory/1 -> Memory1/1, Mux/5
  Memory1/1 -> Mux/4, Memory2/1
  Memory2/1 -> Mux/3, Memory3/1
  Memory4/1 -> Mux/1
  In/1 -> Memory/1
  Mux/1 -> Out/1

== system VEHICLE_DYN_TRAIN/Vehicle System/Vehicle System/Hydraulic brake ==
  note: kPa
  note: Pa
  note: Pmc
  note: vacuum booster output
  Brake command : Inport
  Abs : Abs
  Add : Sum  Inputs=+--
  Add1 : Sum  Inputs=+-
  Add2 : Sum  Inputs=+-
  Area of master cylinder : Constant  Value=A_mc
  Divide : Product  Inputs=*/
  Gain : Gain  Gain=K_vb
  Gain1 : Gain  Gain=10^3
  Gain2 : Gain  Gain=P_gain
  Integrator : Integrator  ExternalReset=either
  Look-Up Table : Lookup  InputValues=brake_V  Table=brake_Pw  SaturateOnIntegerOverflow=on
  Mastercylinder spring pre-load : Constant  Value=F_cs
  Po : Constant  Value=P_0
  Product : Product  Inputs=3
  Seal friction : Constant  Value=F_cf
  Sign : Signum
  Sqrt : Sqrt  SaturateOnIntegerOverflow=on
  Switch : Switch  Criteria=u2 > Threshold  SaturateOnIntegerOverflow=on  InputSameDT=on
  effective flow coefficient : Constant  Value=C_q
  zero : Constant  Value=0
  Brake torque : Outport  VectorParamsAs1DForOutWhenUnconnected=off
  wires:
  Brake command/1 -> Switch/2, Integrator/2, Gain/1
  Gain/1 -> Add/1
  Mastercylinder spring pre-load/1 -> Add/2
  Seal friction/1 -> Add/3
  Add/1 -> Divide/1
  Area of master cylinder/1 -> Divide/2
  Divide/1 -> Add1/1
  Add1/1 -> Gain1/1
  Abs/1 -> Sqrt/1
  Sqrt/1 -> Product/1
  Sign/1 -> Product/2
  effective flow coefficient/1 -> Product/3
  Gain1/1 -> Sign/1, Abs/1
  Look-Up Table/1 -> Add1/2, Add2/1
  Po/1 -> Add2/2
  Add2/1 -> Gain2/1
  Gain2/1 -> Brake torque/1
  Integrator/1 -> Look-Up Table/1
  Switch/1 -> Integrator/1
  Product/1 -> Switch/1
  zero/1 -> Switch/3

== system VEHICLE_DYN_TRAIN/Vehicle System/Vehicle System/Powertrain1 ==
  w shaft : Inport
  throttle : Inport  Port=2
  Constant : Constant  Value=0
  DIESEL ENGINE : Subsystem
  DRIVELINE : Subsystem
  Terminator1 : Terminator
  T shaft : Outport  VectorParamsAs1DForOutWhenUnconnected=off
  wires:
  throttle/1 -> DIESEL ENGINE/2(driver  demand), DRIVELINE/3(demand)
  w shaft/1 -> DRIVELINE/4(w shaft)
  DRIVELINE/2(T shaft) -> T shaft/1
  DRIVELINE/1(w pump) -> DIESEL ENGINE/1(engine speed)
  DIESEL ENGINE/1(engine torque) -> DRIVELINE/1("T eng ")
  Constant/1 -> DRIVELINE/2(T motor)
  DRIVELINE/3(w motor) -> Terminator1/1
